simulink model "Simulink_VDP_Koopman"  (R2022a)
settings: Solver=FixedStepAuto  StartTime=0.0  StopTime=Tf  FixedStep=Ts  RelTol=1e-3
values from neighbouring files (symbols this model uses):
  D = zeros(size(Z,1),size(U,1))    [VanDerPol_MPC_Koopman.m]
  ss_0 = Spline_Radial_Obs(x_0,X0)    [VanDerPol_MPC_Evaluation.m]
  Ts = 1e-2    (= 0.01)    [VanDerPol_MPC.m]
undefined symbols (not defined in the file or in its folder): A, B
libraries: mpclib x1
settings Model: Creator=sergiovaneg  LastModifiedBy=sergiovaneg

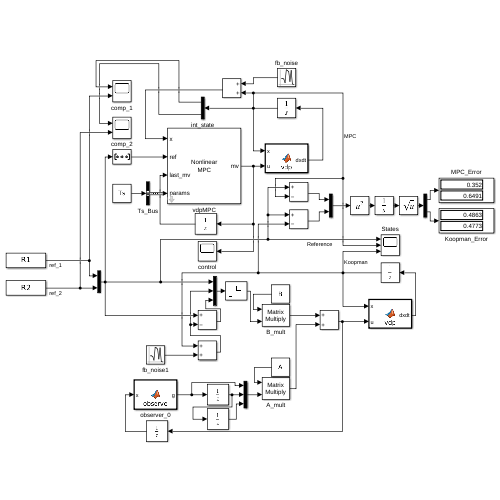
[thumbnail: Simulink's stored preview of the top-level diagram]
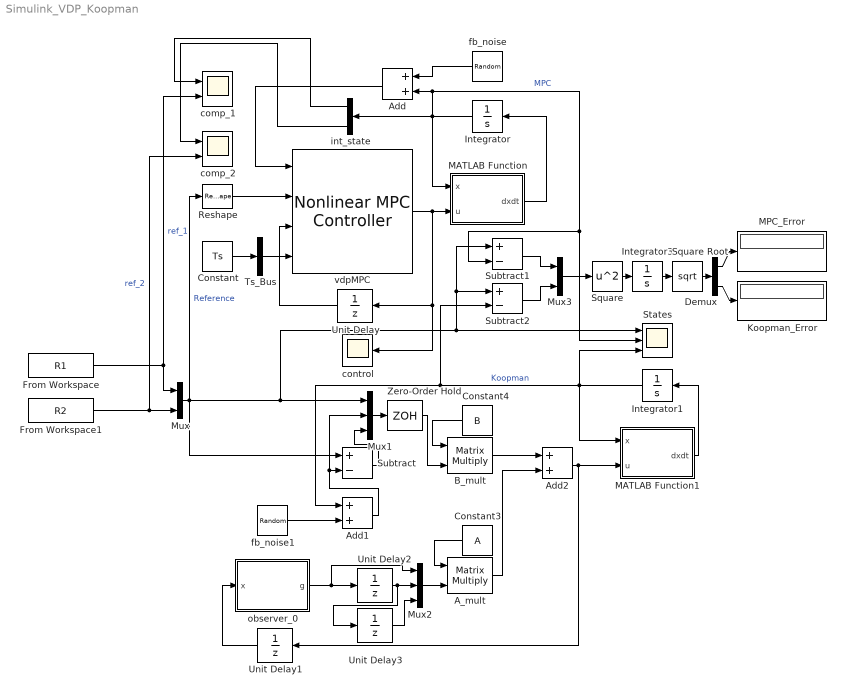
== system Simulink_VDP_Koopman ==
  A_mult : Product  Multiplication=Matrix(*)
  Add : Sum
  Add1 : Sum
  Add2 : Sum
  B_mult : Product  Multiplication=Matrix(*)
  Constant : Constant  Value=Ts
  Constant3 : Constant  Value=A  VectorParams1D=off
  Constant4 : Constant  Value=B  VectorParams1D=off
  Demux : Demux  Outputs=2
  From Workspace : FromWorkspace  VariableName=R1
  From Workspace1 : FromWorkspace  VariableName=R2
  Integrator : Integrator  InitialCondition=[0;0]
  Integrator1 : Integrator  InitialCondition=[0;0]
  Integrator3 : Integrator
  Koopman_Error : Display
  MATLAB Function : MATLAB Function  TreatAsAtomicUnit=on
  MATLAB Function1 : MATLAB Function  TreatAsAtomicUnit=on
  MPC_Error : Display
      settings: Decimation=3
  Mux : Mux  Inputs=2
  Mux1 : Mux  Inputs=3
  Mux2 : Mux  Inputs=3
  Mux3 : Mux  Inputs=2
  Reshape : Reshape  OutputDimensionality=Row vector (2-D)
  Square : Math  Operator=square
  Square Root : Sqrt
  States : Scope  NumInputPorts=3
  Subtract : Sum  Inputs=+-
  Subtract1 : Sum  Inputs=+-
  Subtract2 : Sum  Inputs=+-
  Ts_Bus : BusCreator  Inputs=1  OutDataTypeStr=Bus: Ts_Bus  NonVirtualBus=on
      settings: InheritFromInputs=off
  Unit Delay : UnitDelay  SampleTime=-1  HasFrameUpgradeWarning=on
  Unit Delay1 : UnitDelay  SampleTime=Ts  HasFrameUpgradeWarning=on
  Unit Delay2 : UnitDelay  InitialCondition=ss_0  SampleTime=-1  HasFrameUpgradeWarning=on
  Unit Delay3 : UnitDelay  InitialCondition=ss_0  SampleTime=-1  HasFrameUpgradeWarning=on
  Zero-Order Hold : ZeroOrderHold  SampleTime=-1
  comp_1 : Scope  NumInputPorts=2
  comp_2 : Scope  NumInputPorts=2
  control : Scope
  fb_noise : RandomNumber  Variance=0.001  Seed=[2;3]  SampleTime=Ts
  fb_noise1 : RandomNumber  Variance=0.001  Seed=[2;3]  SampleTime=Ts
  int_state : Demux  Outputs=2
  observer_0 : MATLAB Function  TreatAsAtomicUnit=on
  vdpMPC : mpclib/Nonlinear MPC Controller  nlmpcobj=nlobj  UseObjectTs=on  UseMEX=off  md_enabled=off  mvtarget_enabled=off  param_enabled=on  cost_enabled=off  mvseq_enabled=off  stateseq_enabled=off  ovseq_enabled=off  slack_enabled=off  status_enabled=off  ov_min=off  ov_max=off  mv_min=off  mv_max=off  mvrate_min=off  mvrate_max=off  state_min=off  state_max=off  ov_weight=off  mv_weight=off  mvrate_weight=off  ecr_weight=off  nlp_initialize=off
  wires:
  From Workspace/1 -> Mux/1, comp_1/2  "ref_1"
  Integrator/1 -> Subtract1/2, States/2, Add/2, int_state/1, MATLAB Function/1(x)  "MPC"
  From Workspace1/1 -> comp_2/2, Mux/2  "ref_2"
  Mux/1 -> Subtract/1, Reshape/1, Subtract1/1, Subtract2/1, States/1, Mux1/1  "Reference"
  Integrator1/1 -> States/3, Subtract2/2, Add1/1, MATLAB Function1/1(x)  "Koopman"
  fb_noise/1 -> Add/1
  Add2/1 -> Unit Delay1/1, MATLAB Function1/2(u)
  MATLAB Function/1(dxdt) -> Integrator/1
  vdpMPC/1 -> Unit Delay/1, control/1, MATLAB Function/2(u)
  MATLAB Function1/1(dxdt) -> Integrator1/1
  Add/1 -> vdpMPC/1
  Constant/1 -> Ts_Bus/1
  A_mult/1 -> Add2/2
  Constant4/1 -> B_mult/1
  Constant3/1 -> A_mult/1
  Unit Delay/1 -> vdpMPC/3
  Zero-Order Hold/1 -> B_mult/2
  B_mult/1 -> Add2/1
  Add1/1 -> Mux1/2, Subtract/2
  Reshape/1 -> vdpMPC/2
  Unit Delay1/1 -> observer_0/1(x)
  Ts_Bus/1 -> vdpMPC/4
  int_state/1 -> comp_1/1
  int_state/2 -> comp_2/1
  fb_noise1/1 -> Add1/2
  Mux1/1 -> Zero-Order Hold/1
  Subtract/1 -> Mux1/3
  observer_0/1(g) -> Unit Delay2/1, Mux2/1
  Unit Delay2/1 -> Unit Delay3/1, Mux2/2
  Unit Delay3/1 -> Mux2/3
  Subtract1/1 -> Mux3/1
  Subtract2/1 -> Mux3/2
  Mux3/1 -> Square/1
  Square/1 -> Integrator3/1
  Integrator3/1 -> Square Root/1
  Square Root/1 -> Demux/1
  Demux/1 -> MPC_Error/1
  Demux/2 -> Koopman_Error/1
  Mux2/1 -> A_mult/2

== matlab function Simulink_VDP_Koopman/MATLAB Function ==
  data: x input; u input; dxdt output
function dxdt = vdp(x,u)
    dxdt = zeros(2,1);
    dxdt(1) = 2*x(2);
    dxdt(2) = -0.8*x(1)+2*x(2)-10*(x(1)^2)*x(2)+u;

== matlab function Simulink_VDP_Koopman/observer_0 ==
  data: x input; g output; X0 parameter
function g = observe(x,X0)
    g=zeros(size(x,1)+size(X0,2),1);
    aux = vecnorm(X0-x)';
    g(1:size(x,1))=x;
    g(size(x,1)+1:end)=aux.*log(aux.^aux);
end

== matlab function Simulink_VDP_Koopman/MATLAB Function1 ==
  data: x input; u input; dxdt output
function dxdt = vdp(x,u)
    dxdt = zeros(2,1);
    dxdt(1) = 2*x(2);
    dxdt(2) = -0.8*x(1)+2*x(2)-10*(x(1)^2)*x(2)+u;
